simulink model "headway_controller_pd_test"  (R2020b)
settings: Solver=VariableStepAuto  StartTime=0.0  StopTime=500  RelTol=1e-3
libraries: pid_lib x1, simulink x1
settings Model: Creator=anime  LastModifiedBy=anime

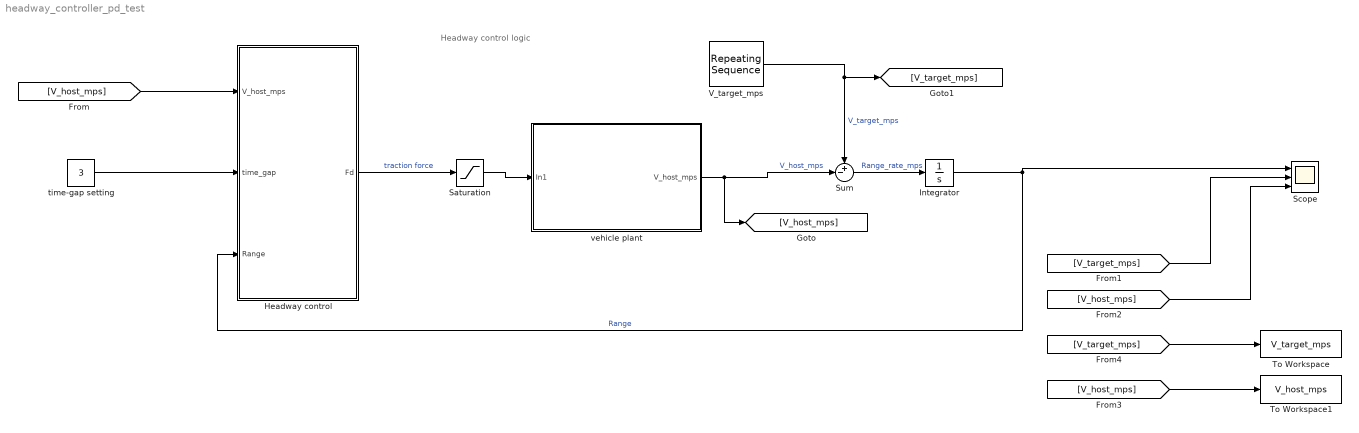
== system headway_controller_pd_test ==
  note: Headway control logic
  Headway control : Subsystem
  Integrator : Integrator
  Saturation : Saturate  UpperLimit=1000  LowerLimit=-1000
  Scope : Scope  NumInputPorts=3
  Sum : Sum  Inputs=+-|
  To Workspace : ToWorkspace  VariableName=V_target_mps  SampleTime=-1
  To Workspace1 : ToWorkspace  VariableName=V_host_mps  SampleTime=-1
  "V_target_mps " : simulink/Sources/Repeating Sequence  rep_seq_t=[0 150 250 350 600]  rep_seq_y=[32 22 22 28 28]
  time-gap setting : Constant  Value=3
  vehicle plant : Subsystem
  wires:
  time-gap setting/1 -> Headway control/2(time_gap)
  Headway control/1(Fd) -> Saturation/1  "traction force"
  Saturation/1 -> vehicle plant/1(In1)
  vehicle plant/1(V_host_mps) -> [V_host_mps], Sum/2  "V_host_mps"
  Sum/1 -> Integrator/1  "Range_rate_mps"
  Integrator/1 -> Headway control/3(Range), Scope/1  "Range"
  "V_target_mps "/1 -> Sum/1, [V_target_mps]  "V_target_mps"
  [V_host_mps] -> Headway control/1(V_host_mps)
  [V_target_mps] -> Scope/2
  [V_host_mps] -> Scope/3
  [V_host_mps] -> To Workspace1/1
  [V_target_mps] -> To Workspace/1

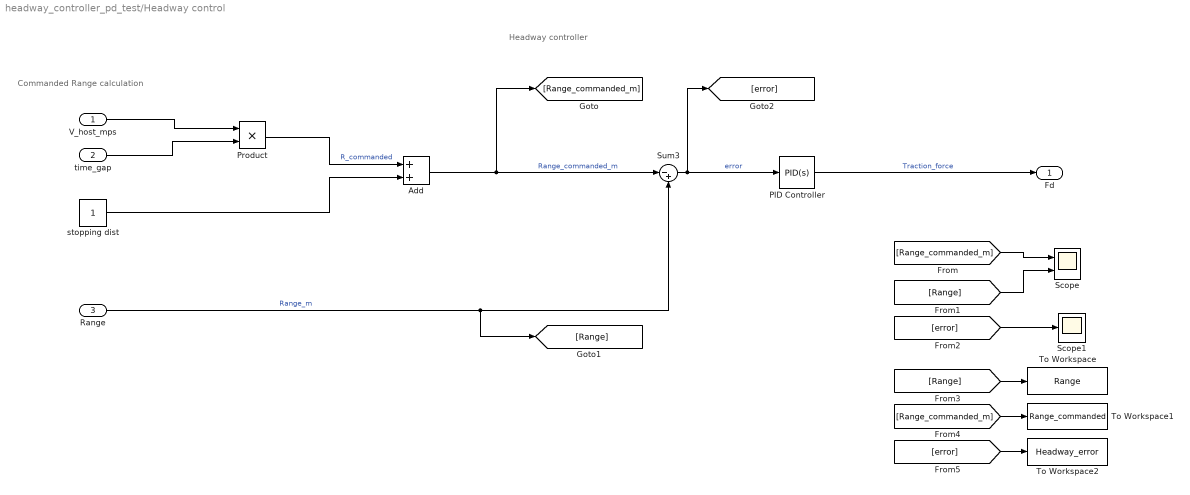
== system headway_controller_pd_test/Headway control ==
  note: Headway controller
  note: Commanded Range calculation
  V_host_mps : Inport
  time_gap : Inport  Port=2
  Range : Inport  Port=3
  Add : Sum
  PID Controller : pid_lib/PID Controller  Controller=PID  Form=Parallel  TimeDomain=Continuous-time  UseExternalTs=off  SampleTime=-1  IntegratorMethod=Forward Euler  FilterMethod=Forward Euler  ControllerParametersSource=internal  P=100  I=3  D=950  UseFilter=on  N=75  TunerSelectOption=Transfer Function Based (PID Tuner App)  InitialConditionSource=internal  InitialConditionForIntegrator=0  InitialConditionForFilter=0  DifferentiatorICPrevScaledInput=0  ExternalReset=none  TrackingMode=off  Kt=1  LimitOutput=off  SatLimitsSource=internal  UpperSaturationLimit=inf  LowerSaturationLimit=-inf  LinearizeAsGain=on  AntiWindupMode=none  Kb=1  POutMin=[]  POutMax=[]  IOutMin=[]  IOutMax=[]  DOutMin=[]  DOutMax=[]  NOutMin=[]  NOutMax=[]  SumOutMin=[]  SumOutMax=[]  SaturationOutMin=[]  SaturationOutMax=[]  PParamMin=[]  PParamMax=[]  IParamMin=[]  IParamMax=[]  DParamMin=[]  DParamMax=[]  NParamMin=[]  NParamMax=[]  KbParamMin=[]  KbParamMax=[]  KtParamMin=[]  KtParamMax=[]  KbOutMin=[]  KbOutMax=[]  KtOutMin=[]  KtOutMax=[]  IntegratorOutMin=[]  IntegratorOutMax=[]  FilterOutMin=[]  FilterOutMax=[]  SumI1OutMin=[]  SumI1OutMax=[]  SumI2OutMin=[]  SumI2OutMax=[]  SumI3OutMin=[]  SumI3OutMax=[]  SumI4OutMin=[]  SumI4OutMax=[]  SumDOutMin=[]  SumDOutMax=[]  DifferentiatorOutMin=[]  DifferentiatorOutMax=[]  FilterDiffOutCoefMin=[]  FilterDiffOutCoefMax=[]  ReciprocalOutMin=[]  ReciprocalOutMax=[]  SumDenOutMin=[]  SumDenOutMax=[]  SumNumOutMin=[]  SumNumOutMax=[]  DivideOutMin=[]  DivideOutMax=[]  UdiffTsProdOutMin=[]  UdiffTsProdOutMax=[]  NTsProdOutMin=[]  NTsProdOutMax=[]  UintegralTsProdOutMin=[]  UintegralTsProdOutMax=[]  UngainTsProdOutMin=[]  UngainTsProdOutMax=[]  IntegratorContinuousStateAttributes=''  IntegratorStateMustResolveToSignalObject=off  IntegratorRTWStateStorageClass=Auto  FilterContinuousStateAttributes=''  FilterStateMustResolveToSignalObject=off  FilterRTWStateStorageClass=Auto  ParallelPVariant=InternalParameters  IdealPVariant=Disabled  IVariant=InternalParameters  DVariant=InternalParameters  IntegratorVariant=Continuous  SatVariant=Disabled  AWVariant=Passthrough  PCopyVariant=Disabled  TRVariant=Disabled  FdbkBlocksVariant=Forward  IdealPFdbkVariant=Disabled  SatFdbkVariant=Disabled  DerivativeFilterVariant=ContFilter  NVariant=InternalParameters  NCopyVariant=Disabled  FilterICVariant=InternalICsFilter  IntegratorICVariant=InternalICs  ExternalResetVariant=Disabled  TRSumVariant=Passthrough  SumFdbkVariant=Disabled  SumVariant=Sum_PID  TsampFilterVariant=InternalTs  TsampNgainVariant=Passthrough  TsampIntegralVariant=Passthrough  ExternalSaturationOutDataTypeStr=Inherit: Same as second input
  Product : Product
  Scope : Scope  NumInputPorts=2
  Scope1 : Scope
  Sum3 : Sum  Inputs=|-+
  To Workspace : ToWorkspace  VariableName=Range  SampleTime=-1
  To Workspace1 : ToWorkspace  VariableName=Range_commanded  SampleTime=-1
  To Workspace2 : ToWorkspace  VariableName=Headway_error  SampleTime=-1
  stopping dist : Constant
  Fd : Outport
  wires:
  Sum3/1 -> [error], PID Controller/1  "error"
  Range/1 -> [Range], Sum3/2  "Range_m"
  Add/1 -> [Range_commanded_m], Sum3/1  "Range_commanded_m"
  stopping dist/1 -> Add/2
  Product/1 -> Add/1  "R_commanded"
  time_gap/1 -> Product/2
  PID Controller/1 -> Fd/1  "Traction_force"
  V_host_mps/1 -> Product/1
  [Range_commanded_m] -> Scope/1
  [Range] -> Scope/2
  [Range] -> To Workspace/1
  [Range_commanded_m] -> To Workspace1/1
  [error] -> To Workspace2/1
  [error] -> Scope1/1

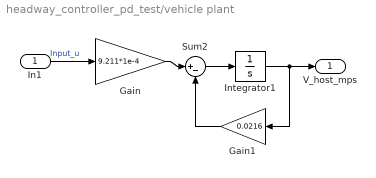
== system headway_controller_pd_test/vehicle plant ==
  In1 : Inport
  Gain : Gain  Gain=9.211*1e-4
  Gain1 : Gain  Gain=0.0216
  Integrator1 : Integrator  InitialCondition=25
  Sum2 : Sum  Inputs=|+-
  V_host_mps : Outport  VectorParamsAs1DForOutWhenUnconnected=off
  wires:
  Sum2/1 -> Integrator1/1
  In1/1 -> Gain/1  "Input_u"
  Gain1/1 -> Sum2/2
  Integrator1/1 -> V_host_mps/1, Gain1/1
  Gain/1 -> Sum2/1
